simulink model "Lab1_8B"  (R2018a)
settings: Solver=VariableStepAuto  StartTime=0.0  StopTime=3  RelTol=1e-6
settings Model: Creator=melab2  LastModifiedBy=rahul

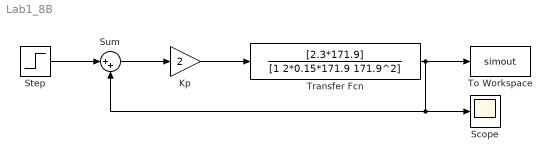
== system Lab1_8B ==
  Kp : Gain  Gain=2
  Scope : Scope
  Step : Step  SampleTime=0
  Sum : Sum  Inputs=|++
  To Workspace : ToWorkspace  VariableName=simout  SampleTime=-1
  Transfer Fcn : TransferFcn  Numerator=[2.3*171.9]  Denominator=[1 2*0.15*171.9 171.9^2]
  wires:
  Kp/1 -> Transfer Fcn/1
  Sum/1 -> Kp/1
  Transfer Fcn/1 -> Sum/2, Scope/1, To Workspace/1
  Step/1 -> Sum/1
